simulink model "Q5"  (R2025a)
settings: Solver=VariableStepAuto  StartTime=0.0  StopTime=5  RelTol=1e-3
settings Model: Creator=64892  LastModifiedBy=64892

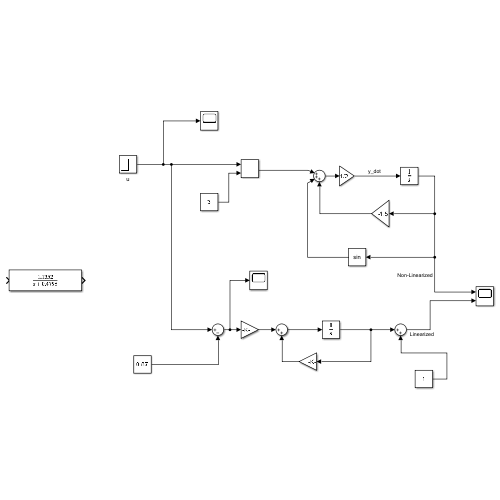
[thumbnail: Simulink's stored preview of the top-level diagram]
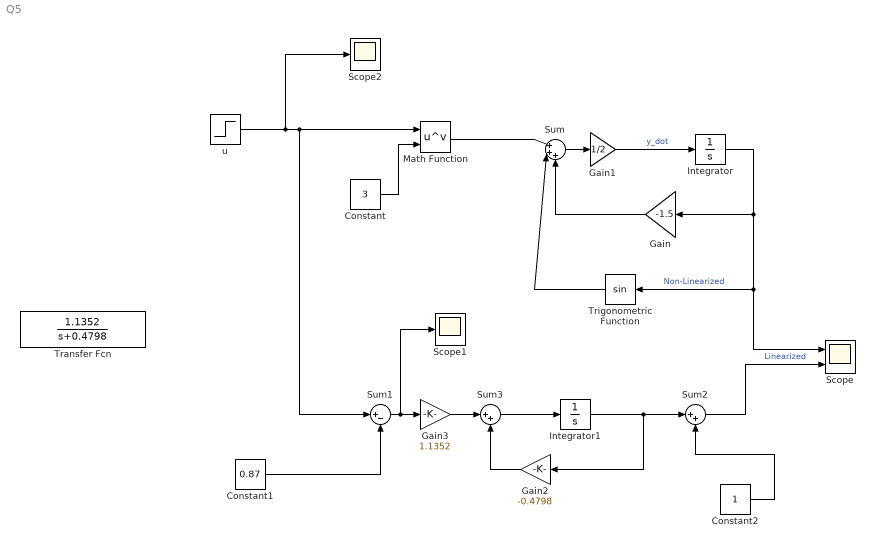
== system Q5 ==
  Constant : Constant  Value=3
  Constant1 : Constant  Value=0.87
  Constant2 : Constant
  Gain : Gain  Gain=-1.5
  Gain1 : Gain  Gain=1/2
  Gain2 : Gain  Gain=-0.4798
  Gain3 : Gain  Gain=1.1352
  Integrator : Integrator
  Integrator1 : Integrator  InitialCondition=-1
  Math Function : Math  Operator=pow
  Scope : Scope  NumInputPorts=2
      settings: ActiveDisplayYMinimum=0  ActiveDisplayYMaximum=2
  Scope1 : Scope
      settings: ActiveDisplayYMinimum=-1  ActiveDisplayYMaximum=1
  Scope2 : Scope
      settings: ActiveDisplayYMinimum=-1  ActiveDisplayYMaximum=1  DataLoggingVariableName=ScopeData2
  Sum : Sum  Inputs=|+++
  Sum1 : Sum  Inputs=|+-
  Sum2 : Sum  Inputs=|++
  Sum3 : Sum  Inputs=|++
  Transfer Fcn : TransferFcn  Numerator=[1.1352]  Denominator=[1 0.4798]
  Trigonometric Function : Trigonometry
  u : Step  Time=0  Before=1  SampleTime=0
  wires:
  Integrator/1 -> Scope/1, Trigonometric Function/1, Gain/1  "Non-Linearized"
  u/1 -> Scope2/1, Sum1/1, Math Function/1
  Constant/1 -> Math Function/2
  Math Function/1 -> Sum/1
  Sum/1 -> Gain1/1
  Gain1/1 -> Integrator/1  "y_dot"
  Gain/1 -> Sum/3
  Trigonometric Function/1 -> Sum/2
  Constant1/1 -> Sum1/2
  Sum2/1 -> Scope/2  "Linearized"
  Constant2/1 -> Sum2/2
  Sum1/1 -> Gain3/1, Scope1/1
  Sum3/1 -> Integrator1/1
  Gain2/1 -> Sum3/2
  Gain3/1 -> Sum3/1
  Integrator1/1 -> Gain2/1, Sum2/1
